simulink model "LQR_Control"  (R2024a)
settings: Solver=VariableStepAuto  StartTime=0.0  StopTime=100  RelTol=1e-3
values from neighbouring files (symbols this model uses):
  a = 0.056/2    (= 0.028)    [param.m]
  g = 9.81    [param.m]
  Ig = K(5)    [CREOM.m]
  Jp = 7.669e-4    (= 0.0007669)    [param.m]
  Jw = 1.133e-5    (= 1.133e-05)    [param.m]
  K = Kpt + Kpr + Kwt + Kwr    [CREOM.m]
  l = 0.0426    [param.m]
  Mp = 0.263    [param.m]
  Mw = 0.028    [param.m]
  u_1 = 0    [param.m]
  u_2 = 0    [param.m]
  u_3 = 0.01    [param.m]
  u_4 = 0.02    [param.m]
  x0 = [0.1, 0, 0.03, 0]    [param.m]
settings Model: Creator=keita  LastModifiedBy=keita
settings DebuggingCC: UnderSpecifiedDimensionMsg=warning

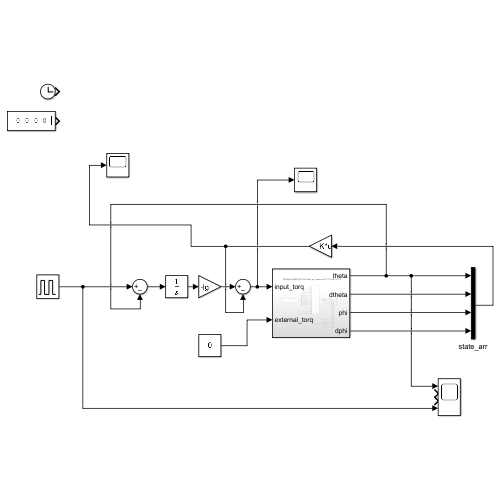
[thumbnail: Simulink's stored preview of the top-level diagram]
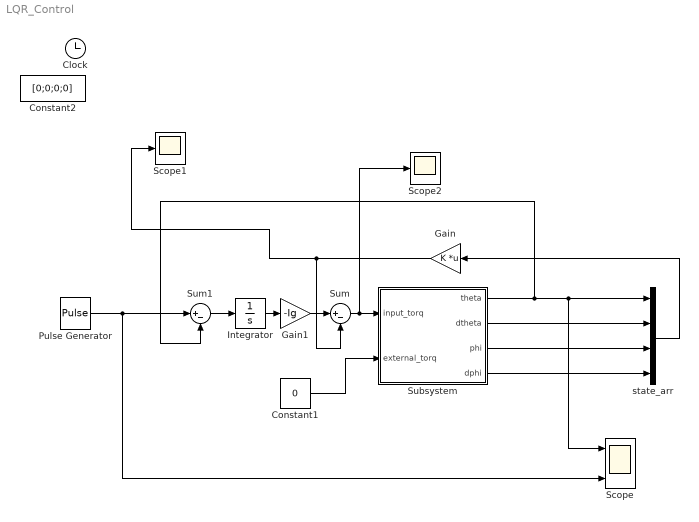
== system LQR_Control ==
  Clock : Clock
  Constant1 : Constant  Value=0
  Constant2 : Constant  Value=[0;0;0;0]
  Gain : Gain  Gain=K  Multiplication=Matrix(K*u)
  Gain1 : Gain  Gain=-Ig
  Integrator : Integrator
  Pulse Generator : DiscretePulseGenerator  PulseType=Time based  Amplitude=0.05  Period=10  PulseWidth=30
  Scope : Scope  NumInputPorts=4
  Scope1 : Scope
  Scope2 : Scope
  Subsystem : Subsystem
  Sum : Sum  Inputs=|+-
  Sum1 : Sum  Inputs=|+-
  state_arr : Mux
  wires:
  Subsystem/1(theta) -> state_arr/1, Scope/1, Sum1/2
  Subsystem/3(phi) -> state_arr/3
  Subsystem/4(dphi) -> state_arr/4
  Gain/1 -> Scope1/1, Sum/2
  Sum/1 -> Scope2/1, Subsystem/1(input_torq)
  state_arr/1 -> Gain/1
  Sum1/1 -> Integrator/1
  Integrator/1 -> Gain1/1
  Gain1/1 -> Sum/1
  Constant1/1 -> Subsystem/2(external_torq)
  Pulse Generator/1 -> Scope/4, Sum1/1
  Subsystem/2(dtheta) -> state_arr/2

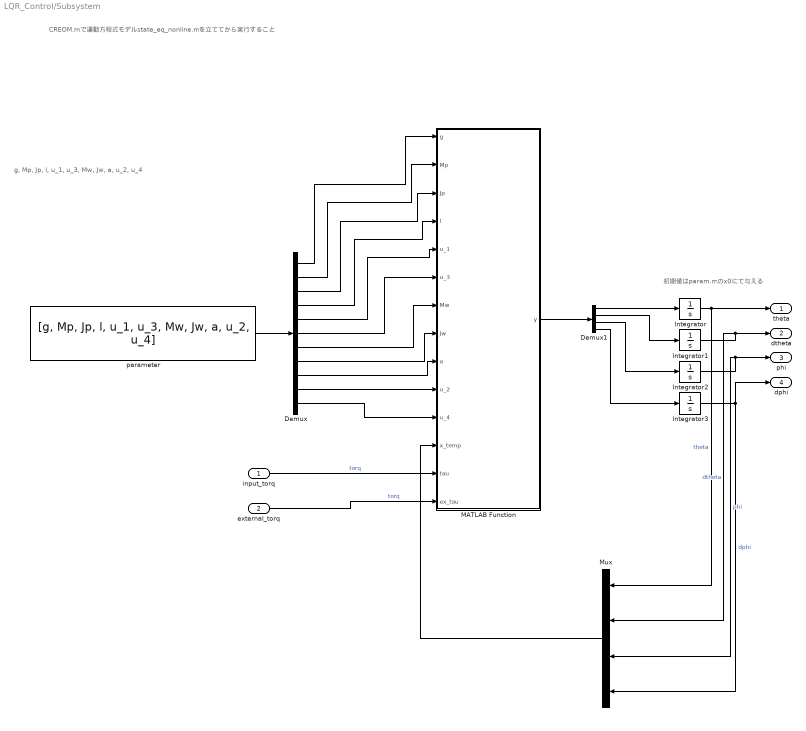
== system LQR_Control/Subsystem ==
  note: 初期値はparam.mのx0にて与える
  note: CREOM.mで運動方程式モデルstate_eq_nonline.mを立ててから実行すること
  note: g, Mp, Jp, l, u_1, u_3, Mw, Jw, a, u_2, u_4
  input_torq : Inport
  external_torq : Inport  Port=2
  Demux : Demux  Outputs=11
  Demux1 : Demux
  Integrator : Integrator  InitialCondition=x0(1)
  Integrator1 : Integrator  InitialCondition=x0(2)
  Integrator2 : Integrator  InitialCondition=x0(3)
  Integrator3 : Integrator  InitialCondition=x0(4)
  MATLAB Function : MATLAB Function  TreatAsAtomicUnit=on
  Mux : Mux
  parameter : Constant  Value=[g, Mp, Jp, l, u_1, u_3, Mw, Jw, a, u_2, u_4]
  theta : Outport
  dtheta : Outport  Port=2
  phi : Outport  Port=3
  dphi : Outport  Port=4
  wires:
  Demux/1 -> MATLAB Function/1(g)
  MATLAB Function/1(y) -> Demux1/1
  Demux1/2 -> Integrator1/1
  Demux/4 -> MATLAB Function/4(l)
  Demux1/3 -> Integrator2/1
  Demux1/4 -> Integrator3/1
  Integrator2/1 -> phi/1, Mux/3  "phi"
  Integrator3/1 -> Mux/4, dphi/1  "dphi"
  Integrator/1 -> theta/1, Mux/1  "theta"
  Integrator1/1 -> dtheta/1, Mux/2  "dtheta"
  Demux/5 -> MATLAB Function/5(u_1)
  Demux/8 -> MATLAB Function/8(Jw)
  Demux/9 -> MATLAB Function/9(a)
  Demux1/1 -> Integrator/1
  Demux/3 -> MATLAB Function/3(Jp)
  Demux/2 -> MATLAB Function/2(Mp)
  parameter/1 -> Demux/1
  Demux/11 -> MATLAB Function/11(u_4)
  Demux/10 -> MATLAB Function/10(u_2)
  Demux/6 -> MATLAB Function/6(u_3)
  Demux/7 -> MATLAB Function/7(Mw)
  input_torq/1 -> MATLAB Function/13(tau)  "torq"
  external_torq/1 -> MATLAB Function/14(ex_tau)  "torq"
  Mux/1 -> MATLAB Function/12(x_temp)

== matlab function LQR_Control/Subsystem/MATLAB Function ==
  data: g input; y output; Mp input; Jp input; l input; u_1 input; u_3 input; Mw input; Jw input; a input; u_2 input; u_4 input; x_temp input; tau input; ex_tau input
function y = NLM( g, Mp, Jp, l, u_1, u_3, Mw, Jw, a, u_2, u_4, x_temp, tau, ex_tau)
y = zeros(4,1);
y = state_eq_nonline(g, Mp, Jp, l, u_1, u_3, Mw, Jw, a, u_2, u_4, x_temp, tau,ex_tau);

end
